simulink model "IO_FBL"  (R2023b)
settings: Solver=VariableStepAuto  StartTime=0.0  StopTime=60  RelTol=1e-6
values from neighbouring files (symbols this model uses):
  A = Ixx-Kpdot    (= 4100300)    [ShipFinStabilizers.m]
  b = B/A    (= -0.123183501573)    [ShipFinStabilizers.m]    (also in analisi_LUCIA.m = 1)
  B = Kp + Kup - 2*Kalpha*rf/U    (= -505089.3115)    [ShipFinStabilizers.m]
  c = C/A    (= -0.101455991025)    [ShipFinStabilizers.m]
  C = Knl    (= -416000)    [ShipFinStabilizers.m]
  d = D/A    (= -0.0647513596566)    [ShipFinStabilizers.m]    (also in analisi_LUCIA.m = -0.1)
  D = KphiUU*U^2    (= -265500)    [ShipFinStabilizers.m]
  f = F/A    (= -0.00439842816379)    [ShipFinStabilizers.m]
  F = -2*Kalpha    (= -18034.875)    [ShipFinStabilizers.m]
  Fw = 0.2    [ShipFinStabilizers.m]    (also in plotRoutine.m = Fw_vect(i))
  omega_w = 1.3    [ShipFinStabilizers.m]    (also in plotRoutine.m = omega_w_vect(j))
  sat = 45    [ShipFinStabilizers.m]
  x0 = [deg2rad(20);0]    [ShipFinStabilizers.m]
settings Model: Creator=valen  LastModifiedBy=valen

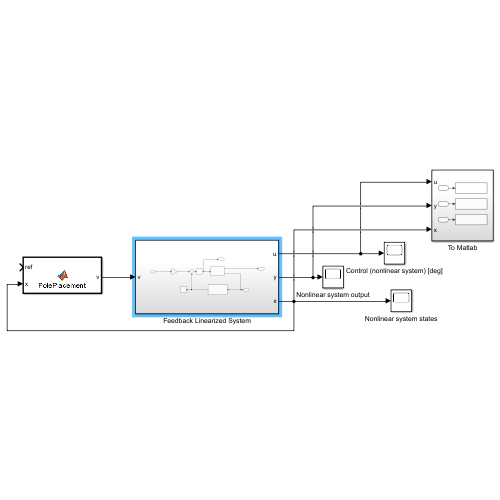
[thumbnail: Simulink's stored preview of the top-level diagram]
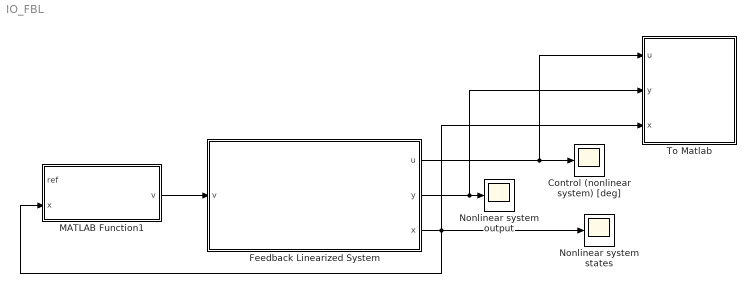
== system IO_FBL ==
  Control (nonlinear system) [deg] : Scope
  Feedback Linearized System : Subsystem
  MATLAB Function1 : MATLAB Function  TreatAsAtomicUnit=on
  Nonlinear system output : Scope
  Nonlinear system states : Scope
  To Matlab : Subsystem
  wires:
  Feedback Linearized System/3(x) -> To Matlab/3(x), Nonlinear system states/1, MATLAB Function1/2(x)
  MATLAB Function1/1(v) -> Feedback Linearized System/1(v)
  Feedback Linearized System/2(y) -> To Matlab/2(y), Nonlinear system output/1
  Feedback Linearized System/1(u) -> To Matlab/1(u), Control (nonlinear system) [deg]/1

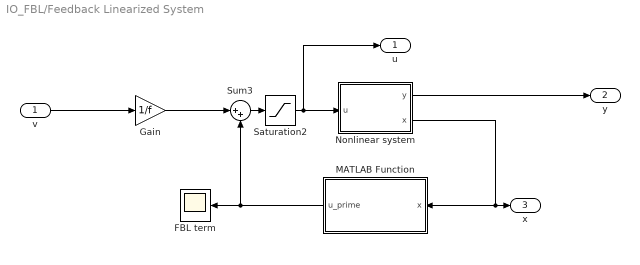
== system IO_FBL/Feedback Linearized System ==
  v : Inport
  FBL term : Scope
  Gain : Gain  Gain=1/f
  MATLAB Function : MATLAB Function  TreatAsAtomicUnit=on
  Nonlinear system : Subsystem
  Saturation2 : Saturate  UpperLimit=sat  LowerLimit=-sat
  Sum3 : Sum  Inputs=|++
  u : Outport
  y : Outport  Port=2
  x : Outport  Port=3
  wires:
  Sum3/1 -> Saturation2/1
  Saturation2/1 -> Nonlinear system/1(u), u/1
  Gain/1 -> Sum3/1
  Nonlinear system/2(x) -> MATLAB Function/1(x), x/1
  MATLAB Function/1(u_prime) -> FBL term/1, Sum3/2
  Nonlinear system/1(y) -> y/1
  v/1 -> Gain/1

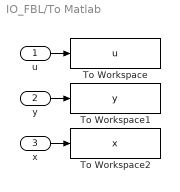
== system IO_FBL/To Matlab ==
  u : Inport
  y : Inport  Port=2
  x : Inport  Port=3
  To Workspace : ToWorkspace  VariableName=u  SaveFormat=Structure With Time  SampleTime=-1
  To Workspace1 : ToWorkspace  VariableName=y  SaveFormat=Structure With Time  SampleTime=-1
  To Workspace2 : ToWorkspace  VariableName=x  SaveFormat=Structure With Time  SampleTime=-1
  wires:
  y/1 -> To Workspace1/1
  x/1 -> To Workspace2/1
  u/1 -> To Workspace/1

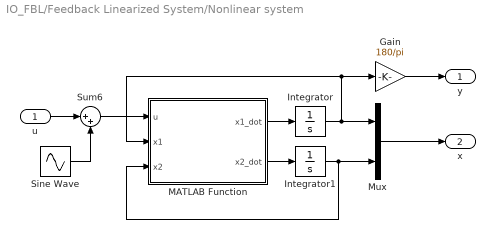
== system IO_FBL/Feedback Linearized System/Nonlinear system ==
  u : Inport
  Gain : Gain  Gain=180/pi
  Integrator : Integrator  InitialCondition=x0(1)
  Integrator1 : Integrator  InitialCondition=x0(2)
  MATLAB Function : MATLAB Function  TreatAsAtomicUnit=on
  Mux : Mux  Inputs=2
  Sine Wave : Sin  Amplitude=Fw/F*A  Frequency=omega_w  SampleTime=0
  Sum6 : Sum  Inputs=|++
  y : Outport  PortDimensions=1
  x : Outport  Port=2
  wires:
  Integrator1/1 -> Mux/2, MATLAB Function/3(x2)
  Integrator/1 -> Mux/1, Gain/1, MATLAB Function/2(x1)
  MATLAB Function/2(x2_dot) -> Integrator1/1
  MATLAB Function/1(x1_dot) -> Integrator/1
  Mux/1 -> x/1
  Sine Wave/1 -> Sum6/2
  u/1 -> Sum6/1
  Sum6/1 -> MATLAB Function/1(u)
  Gain/1 -> y/1

== matlab function IO_FBL/Feedback Linearized System/Nonlinear system/MATLAB Function ==
  data: u input; x1_dot output; x1 input; x2 input; x2_dot output; A parameter; B parameter; C parameter; D parameter; E parameter; F parameter
function [x1_dot,x2_dot] = ship(u,x1,x2, A, B, C, D, E, F)

    x1_dot = x2;
    x2_dot = 1/A*( B*x2 + C*x2*abs(x2) + D*x1 + E*sin(x1) + F*u);

== matlab function IO_FBL/Feedback Linearized System/MATLAB Function ==
  data: x input; u_prime output; b parameter; c parameter; d parameter; e parameter; f parameter
function u_prime = fbl(x,b, c, d, e, f)

    u_prime = 1/f*(-b*x(2) -c*x(2)*abs(x(2)) - d*x(1) - e*sin(x(1)));

end

== matlab function IO_FBL/MATLAB Function1 ==
  data: ref input; x input size=[2,1]; v output
function v = PolePlacement(ref,x)

v = -0.5*x(1) - 1*x(2);
%v = -10*x(1);
